simulink model "FFFBmodel"  (R2022b)
settings: Solver=VariableStepAuto  StartTime=0.0  StopTime=5  MaxStep=0.01  RelTol=1e-3
values from neighbouring files (symbols this model uses):
  dot_x_ref = dot_x(end, :)    [DataEstimationAndConstraints.m]
  friction = friction(:,1:numSample)    [DataReading.m]    (also in DataSampling.m = random(frictionUniformDist, 1, numSample); SensitivityAnalysisConfig.m = 0.5; data.mat = [0.423870600502 0.414714985315 0.508364191084 0.585845302695)
  g = random(gDist, 1, 1)    [DataSampling.m]    (also in SensitivityAnalysisConfig.m = 9.8; data.mat = 9.78798650818)
  PID = [3, 0.5, 0]    [DataEstimationAndConstraints.m]
  u_ref = u    [DataEstimationAndConstraints.m]
  weight = weight(:,1:numSample)    [DataReading.m]    (also in DataSampling.m = random(weightDist, 1, numSample); SensitivityAnalysisConfig.m = 0.025; data.mat = [0.0249399431455 0.0249880813357 0.0249204436802 0.024988815)
libraries: simulink x2, slpidlib x1
settings Model: Creator=w.ar  LastModifiedBy=w.ar

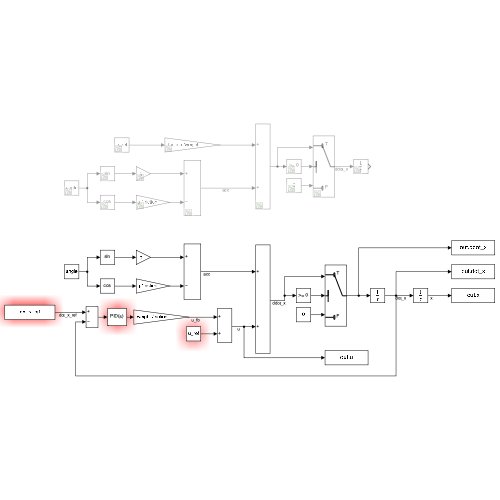
[thumbnail: Simulink's stored preview of the top-level diagram]
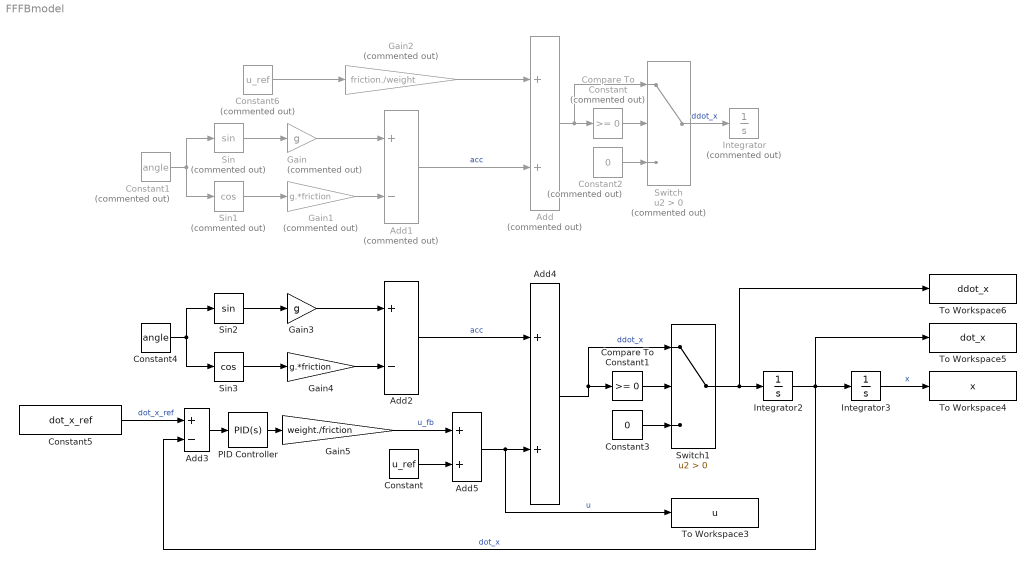
== system FFFBmodel ==
  Add : Sum  Commented=on
  Add1 : Sum  Commented=on  Inputs=+-
  Add2 : Sum  Inputs=+-
  Add3 : Sum  Inputs=+-
  Add4 : Sum
  Add5 : Sum
  Compare To Constant : simulink/Logic and Bit Operations/Compare To Constant  Commented=on  relop=>=  const=0  OutDataTypeStr=boolean
  Compare To Constant1 : simulink/Logic and Bit Operations/Compare To Constant  relop=>=  const=0  OutDataTypeStr=boolean
  Constant : Constant  Value=u_ref
  Constant1 : Constant  Commented=on  Value=angle
  Constant2 : Constant  Commented=on  Value=0
  Constant3 : Constant  Value=0
  Constant4 : Constant  Value=angle
  Constant5 : Constant  Value=dot_x_ref
  Constant6 : Constant  Commented=on  Value=u_ref
  Gain : Gain  Commented=on  Gain=g
  Gain1 : Gain  Commented=on  Gain=g.*friction
  Gain2 : Gain  Commented=on  Gain=friction./weight
  Gain3 : Gain  Gain=g
  Gain4 : Gain  Gain=g.*friction
  Gain5 : Gain  Gain=weight./friction
  Integrator : Integrator  Commented=on
  Integrator2 : Integrator
  Integrator3 : Integrator  UpperSaturationLimit=length
  PID Controller : slpidlib/PID Controller  Controller=PID  Form=Parallel  TimeDomain=Continuous-time  UseExternalTs=off  SampleTime=-1  IntegratorMethod=Forward Euler  FilterMethod=Forward Euler  ControllerParametersSource=internal  P=PID(1)  I=PID(2)  UseKiTs=off  D=PID(3)  N=100  UseFilter=on  TunerSelectOption=Transfer Function Based (PID Tuner App)  InitialConditionSource=internal  InitialConditionForIntegrator=0  InitialConditionForFilter=0  DifferentiatorICPrevScaledInput=0  ExternalReset=none  TrackingMode=off  Kt=1  LimitOutput=off  SatLimitsSource=internal  UpperSaturationLimit=inf  LowerSaturationLimit=-inf  LinearizeAsGain=on  AntiWindupMode=none  Kb=1  LimitIntegrator=off  UpperIntegratorSaturationLimit=inf  LowerIntegratorSaturationLimit=-inf  POutMin=[]  POutMax=[]  IOutMin=[]  IOutMax=[]  DOutMin=[]  DOutMax=[]  NOutMin=[]  NOutMax=[]  SumOutMin=[]  SumOutMax=[]  SaturationOutMin=[]  SaturationOutMax=[]  PParamMin=[]  PParamMax=[]  IParamMin=[]  IParamMax=[]  DParamMin=[]  DParamMax=[]  NParamMin=[]  NParamMax=[]  KbParamMin=[]  KbParamMax=[]  KtParamMin=[]  KtParamMax=[]  KbOutMin=[]  KbOutMax=[]  KtOutMin=[]  KtOutMax=[]  IntegratorOutMin=[]  IntegratorOutMax=[]  FilterOutMin=[]  FilterOutMax=[]  SumI1OutMin=[]  SumI1OutMax=[]  SumI2OutMin=[]  SumI2OutMax=[]  SumI3OutMin=[]  SumI3OutMax=[]  SumI4OutMin=[]  SumI4OutMax=[]  SumDOutMin=[]  SumDOutMax=[]  DifferentiatorOutMin=[]  DifferentiatorOutMax=[]  FilterDiffOutCoefMin=[]  FilterDiffOutCoefMax=[]  ReciprocalOutMin=[]  ReciprocalOutMax=[]  SumDenOutMin=[]  SumDenOutMax=[]  SumNumOutMin=[]  SumNumOutMax=[]  DivideOutMin=[]  DivideOutMax=[]  UdiffTsProdOutMin=[]  UdiffTsProdOutMax=[]  NTsProdOutMin=[]  NTsProdOutMax=[]  UintegralTsProdOutMin=[]  UintegralTsProdOutMax=[]  UngainTsProdOutMin=[]  UngainTsProdOutMax=[]  ClampingZeroOutDataTypeStr=Inherit: Inherit via back propagation  ClampingZeroOutMin=[]  ClampingZeroOutMax=[]  FilterDenConstantOutDataTypeStr=Inherit: Inherit via back propagation  FilterDenConstantOutMin=[]  FilterDenConstantOutMax=[]  PCopyOutDataTypeStr=Inherit: Inherit via back propagation  PCopyOutMin=[]  PCopyOutMax=[]  NCopyOutDataTypeStr=Inherit: Inherit via back propagation  NCopyOutMin=[]  NCopyOutMax=[]  IntegratorContinuousStateAttributes=''  IntegratorStateMustResolveToSignalObject=off  IntegratorRTWStateStorageClass=Auto  FilterContinuousStateAttributes=''  FilterStateMustResolveToSignalObject=off  FilterRTWStateStorageClass=Auto  ParallelPVariant=InternalParameters  IdealPVariant=Disabled  IVariant=InternalParameters  DVariant=InternalParameters  IntegratorVariant=Continuous  SatVariant=Disabled  AWVariant=Passthrough  PCopyVariant=Disabled  TRVariant=Disabled  FdbkBlocksVariant=Forward  IdealPFdbkVariant=Disabled  SatFdbkVariant=Disabled  DerivativeFilterVariant=ContFilter  NVariant=InternalParameters  NCopyVariant=Disabled  FilterICVariant=InternalICsFilter  IntegratorICVariant=InternalICs  ExternalResetVariant=Disabled  TRSumVariant=Passthrough  SumFdbkVariant=Disabled  SumVariant=Sum_PID  TsampFilterVariant=InternalTs  TsampNgainVariant=Passthrough  TsampIntegralVariant=Passthrough  ExternalSaturationOutDataTypeStr=Inherit: Same as second input
  Sin : Trigonometry  Commented=on
  Sin1 : Trigonometry  Commented=on  Operator=cos
  Sin2 : Trigonometry
  Sin3 : Trigonometry  Operator=cos
  Switch : Switch  Commented=on  Criteria=u2 > Threshold  SaturateOnIntegerOverflow=off  InputSameDT=off
  Switch1 : Switch  Criteria=u2 > Threshold  SaturateOnIntegerOverflow=off  InputSameDT=off
  To Workspace3 : ToWorkspace  VariableName=u  SaveFormat=Timeseries  SampleTime=-1
  To Workspace4 : ToWorkspace  VariableName=x  SaveFormat=Timeseries  SampleTime=-1
  To Workspace5 : ToWorkspace  VariableName=dot_x  SaveFormat=Timeseries  SampleTime=-1
  To Workspace6 : ToWorkspace  VariableName=ddot_x  SaveFormat=Timeseries  SampleTime=-1
  wires:
  Sin/1 -> Gain/1
  Add/1 -> Switch/1, Compare To Constant/1
  Constant1/1 -> Sin1/1, Sin/1
  Gain2/1 -> Add/1
  Sin1/1 -> Gain1/1
  Gain1/1 -> Add1/2
  Gain/1 -> Add1/1
  Add1/1 -> Add/2  "acc"
  Constant2/1 -> Switch/3
  Compare To Constant/1 -> Switch/2
  Switch/1 -> Integrator/1  "ddot_x"
  Constant4/1 -> Sin3/1, Sin2/1
  Sin2/1 -> Gain3/1
  Add2/1 -> Add4/1  "acc"
  Integrator2/1 -> Add3/2, To Workspace5/1, Integrator3/1  "dot_x"
  Integrator3/1 -> To Workspace4/1  "x"
  Sin3/1 -> Gain4/1
  Compare To Constant1/1 -> Switch1/2
  Gain4/1 -> Add2/2
  Add3/1 -> PID Controller/1
  Add4/1 -> Switch1/1, Compare To Constant1/1  "ddot_x"
  Gain3/1 -> Add2/1
  Switch1/1 -> To Workspace6/1, Integrator2/1
  PID Controller/1 -> Gain5/1
  Constant3/1 -> Switch1/3
  Constant5/1 -> Add3/1  "dot_x_ref"
  Gain5/1 -> Add5/1  "u_fb"
  Constant/1 -> Add5/2
  Add5/1 -> To Workspace3/1, Add4/2  "u"
  Constant6/1 -> Gain2/1
